simulink model "Mangnorondung"  (R2022b)
settings: Solver=FixedStepAuto  StartTime=0.0  StopTime=150  FixedStep=0.01  RelTol=1e-3
libraries: slpidlib x2
settings Model: Creator=vudin  LastModifiedBy=Acer Nitro
settings SolverCC: ShapePreserveControl=EnableAll  AlgebraicLoopSolver=TrustRegion
settings DataIOCC: ReturnWorkspaceOutputs=off
settings DebuggingCC: UnconnectedInputMsg=warning  UnconnectedOutputMsg=warning  UnconnectedLineMsg=warning  SFMachineParentedDataDiag=warning  ArithmeticOperatorsInVariantConditions=warning
settings ModelReferenceCC: EnableRefExpFcnMdlSchedulingChecks=on
settings SFSimCC: CustomCodeUndefinedFunction=UseInterfaceOnly

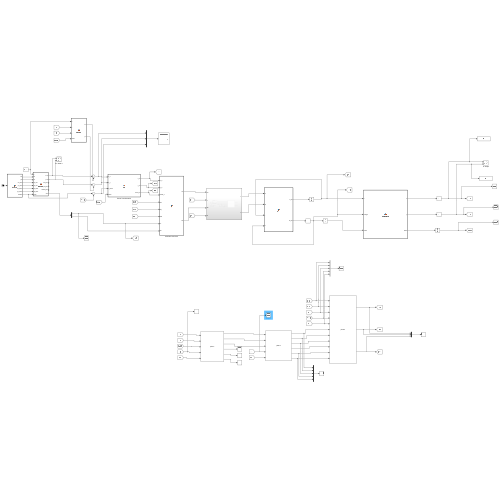
[thumbnail: Simulink's stored preview of the top-level diagram]
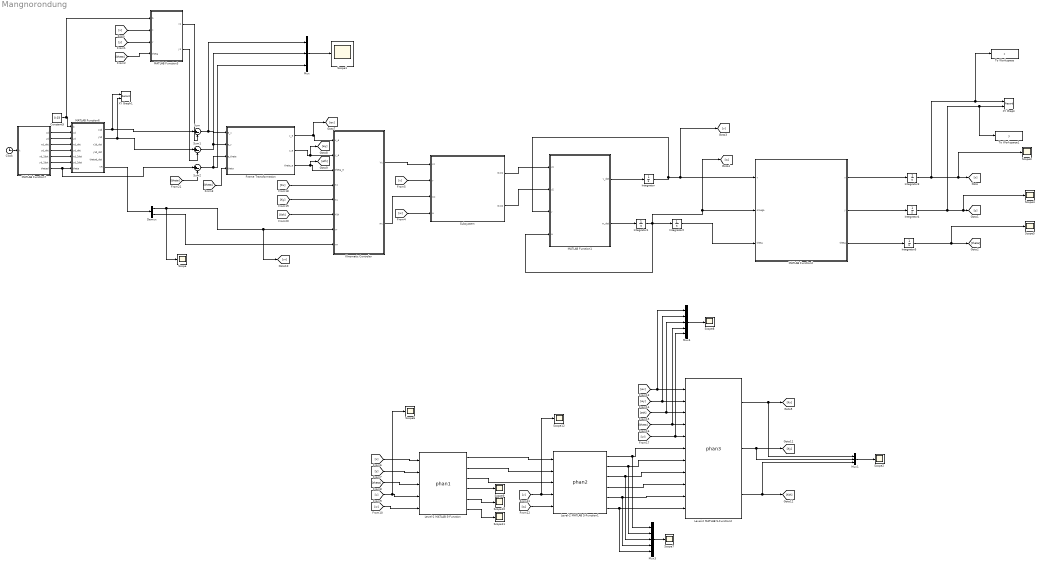
== system Mangnorondung ==
  Clock : Clock
  Constant5 : Constant  Value=0.03
  Demux : Demux  Outputs=2
  Frame Transformation : MATLAB Function  TreatAsAtomicUnit=on
  Integrator{,1..5} (6 alike) : Integrator
  KInematic Controler : MATLAB Function  TreatAsAtomicUnit=on
  Level-2 MATLAB S-Function : M-S-Function  FunctionName=phan1
  Level-2 MATLAB S-Function1 : M-S-Function  FunctionName=phan2
  Level-2 MATLAB S-Function2 : M-S-Function  FunctionName=phan3
  MATLAB Function1 : MATLAB Function  TreatAsAtomicUnit=on
  MATLAB Function2 : MATLAB Function  TreatAsAtomicUnit=on
  MATLAB Function3 : MATLAB Function  TreatAsAtomicUnit=on
  MATLAB Function6 : MATLAB Function  TreatAsAtomicUnit=on
  MATLAB Function7 : MATLAB Function  TreatAsAtomicUnit=on
  Mux : Mux  Inputs=3
  Mux1 : Mux  Inputs=3
  Mux3 : Mux  Inputs=5
  Mux4 : Mux  Inputs=5
  Scope{,1..12} (13 alike) : Scope
  Subsystem : Subsystem
  Sum : Sum  Inputs=|+-
  Sum1 : Sum  Inputs=|+-
  Sum2 : Sum  Inputs=|+-
  To Workspace : ToWorkspace  VariableName=x  SampleTime=-1
  To Workspace1 : ToWorkspace  VariableName=y  SampleTime=-1
  XY Graph : Record  FileSettingsInternal="{\"entries\":[{\"content\":{\"excelSettings\":{\"content\":{},\"type\":\"Streamout.ExcelSettings\"}},\"type\":\"Streamout.FileSettingStorage\",\"uuid\":\"709517b4-b6f2-4336-ad97-cda2d1ea3157\"}],\"packageUris\":[\"http://schema.mathworks.com/mf0/streamout_blocks/R2020a\"],\"version\":\"1.0\"}"  Layout=[1 1]  SignalsInternal="{\"entries\":[{\"content\":{\"signals\":[{\"content\":{\"blockPath\":[\"Mangnorondung/XY Graph\"],\"channel\":[],\"dimensions\":[1],\"domain\":\"Mangnorondung/XY Graph\",\"lineColor\":\"#a2142f\",\"plots\":[1],\"port\":1,\"sid\":[\"\"],\"signalID\":43589,\"signalName\":\"Integrator3\"},\"type\":\"RecordBlkView.Signal\",\"uuid\":\"4f684b5a-924f-486e-9d40-9f936f114ddd\"},{\"content\":{\"blockPath\":[\"Mangnorondung/XY Graph\"],\"channel\":[],\"dimensions\":[1],\"domain\":\"Mangnorondung/XY Graph\",\"lineColor\":\"#139fff\",\"plots\":[1],\"port\":2,\"sid\":[\"\"],\"signalID\":43593,\"signalName\":\"Integrator4\"},\"type\":\"RecordBlkView.Signal\",\"uuid\":\"4d6a86e3-ef4b-4abf-8449-7e6d24bf3609\"}]},\"type\":\"RecordBlkView.InputSignals\",\"uuid\":\"2b587b06-57ab-4d61-b86d-7002576b861b\"}],\"packageUris\":[\"http://schema.mathworks.com/mf0/streamout_blocks/R2020a\"],\"version\":\"1.0\"}"  VisualizationBindings="{\"xyplotplugin\":{\"info\":[{\"series\":[{\"bindingParametersList\":[{\"parameter\":\"X-Axis\",\"signalID\":43589,\"signalName\":\"Integrator3\"},{\"parameter\":\"Y-Axis\",\"signalID\":43593,\"signalName\":\"Integrator4\"}],\"seriesID\":42575}],\"subplotID\":1}]}}"  CompatibilityTag=XY  st=-1
  XY Graph1 : Record  FileSettingsInternal="{\"entries\":[{\"content\":{\"excelSettings\":{\"content\":{},\"type\":\"Streamout.ExcelSettings\"}},\"type\":\"Streamout.FileSettingStorage\",\"uuid\":\"df5eb68b-e3d3-4db8-aae6-13adc78e2c49\"}],\"packageUris\":[\"http://schema.mathworks.com/mf0/streamout_blocks/R2020a\"],\"version\":\"1.0\"}"  Layout=[1 1]  SignalsInternal="{\"entries\":[{\"content\":{\"signals\":[{\"content\":{\"blockPath\":[\"Mangnorondung/XY Graph1\"],\"channel\":[],\"dimensions\":[1],\"domain\":\"Mangnorondung/XY Graph1\",\"lineColor\":\"#a2142f\",\"plots\":[1],\"port\":1,\"sid\":[\"\"],\"signalID\":43597,\"signalName\":\"MATLAB Function6:1\"},\"type\":\"RecordBlkView.Signal\",\"uuid\":\"7454b842-5480-4a32-880b-5852a87a060b\"},{\"content\":{\"blockPath\":[\"Mangnorondung/XY Graph1\"],\"channel\":[],\"dimensions\":[1],\"domain\":\"Mangnorondung/XY Graph1\",\"lineColor\":\"#139fff\",\"plots\":[1],\"port\":2,\"sid\":[\"\"],\"signalID\":43601,\"signalName\":\"MATLAB Function6:2\"},\"type\":\"RecordBlkView.Signal\",\"uuid\":\"a917114d-4933-41c9-b594-8cfc2867815e\"}]},\"type\":\"RecordBlkView.InputSignals\",\"uuid\":\"cfe23017-764e-4c0d-8e92-bd75a684a487\"}],\"packageUris\":[\"http://schema.mathworks.com/mf0/streamout_blocks/R2020a\"],\"version\":\"1.0\"}"  VisualizationBindings="{\"xyplotplugin\":{\"info\":[{\"series\":[{\"bindingParametersList\":[{\"parameter\":\"X-Axis\",\"signalID\":43597,\"signalName\":\"MATLAB Function6:1\"},{\"parameter\":\"Y-Axis\",\"signalID\":43601,\"signalName\":\"MATLAB Function6:2\"}],\"seriesID\":38209}],\"subplotID\":1}]}}"  CompatibilityTag=XY  st=-1
  wires:
  Subsystem/1(Out1) -> MATLAB Function1/1(u1)
  MATLAB Function6/1(x1d) -> XY Graph1/1, Sum/1
  Demux/1 -> Scope/1, [vr], KInematic Controler/7(vr)
  Subsystem/2(Out2) -> MATLAB Function1/2(u2)
  MATLAB Function1/1(v_dot) -> Integrator/1
  MATLAB Function6/6(VR) -> Demux/1
  Mux/1 -> Scope1/1
  MATLAB Function2/3(theta) -> Integrator5/1
  Sum2/1 -> Mux/3, Frame Transformation/3(e_theta)
  Integrator2/1 -> MATLAB Function2/3("theta ")
  MATLAB Function2/1(x) -> Integrator3/1
  Integrator5/1 -> Scope5/1, [theta]
  Integrator1/1 -> [w], MATLAB Function2/2(omega), Integrator2/1, MATLAB Function1/4(w)
  MATLAB Function7/6(yd_2dot) -> MATLAB Function6/7(yd_2dot)
  MATLAB Function7/5(xd_2dot) -> MATLAB Function6/6(xd_2dot)
  Frame Transformation/1(x_e) -> [ex], KInematic Controler/1(x_e)
  [v] -> Subsystem/2(v)
  KInematic Controler/1(Vc) -> Subsystem/1(Vc)
  KInematic Controler/2(wc) -> Subsystem/3(wc)
  MATLAB Function2/2(y) -> Integrator4/1
  Constant5/1 -> MATLAB Function3/1(b), MATLAB Function6/1(b)
  Sum/1 -> Frame Transformation/1(e_x), Mux/1
  MATLAB Function7/1(xd) -> MATLAB Function6/2(xd)
  Demux/2 -> KInematic Controler/8(wr)
  Integrator4/1 -> To Workspace1/1, XY Graph/2, Scope4/1, [y]
  MATLAB Function3/2(y1) -> Sum1/2
  Frame Transformation/2(y_e) -> [ey], KInematic Controler/2(y_e)
  Frame Transformation/3(theta_e) -> [eth], KInematic Controler/3(theta_e)
  [x] -> MATLAB Function3/2(x)
  Integrator3/1 -> To Workspace/1, XY Graph/1, Scope3/1, [x]
  Sum1/1 -> Frame Transformation/2(e_y), Mux/2
  MATLAB Function3/1(x1) -> Sum/2
  Clock/1 -> MATLAB Function7/1(t)
  MATLAB Function7/7(thetad) -> Sum2/1, MATLAB Function6/8(theta)
  [y] -> MATLAB Function3/3(y)
  Integrator/1 -> MATLAB Function1/3(v), [v], MATLAB Function2/1(v)
  MATLAB Function7/4(yd_dot) -> MATLAB Function6/5(yd_dot)
  [theta] -> Frame Transformation/4(theta)
  MATLAB Function7/2(yd) -> MATLAB Function6/3(yd)
  [w] -> Subsystem/4(w)
  MATLAB Function1/2(w_dot) -> Integrator1/1
  MATLAB Function6/2(y1d) -> XY Graph1/2, Sum1/1
  MATLAB Function7/3(xd_dot) -> MATLAB Function6/4(xd_dot)
  Level-2 MATLAB S-Function1/1 -> Mux3/1, Level-2 MATLAB S-Function2/6
  Level-2 MATLAB S-Function1/5 -> Mux3/4, Level-2 MATLAB S-Function2/10
  Level-2 MATLAB S-Function1/3 -> Mux3/3, Level-2 MATLAB S-Function2/8
  Level-2 MATLAB S-Function1/4 -> Level-2 MATLAB S-Function2/9
  Level-2 MATLAB S-Function1/2 -> Mux3/2, Level-2 MATLAB S-Function2/7
  Level-2 MATLAB S-Function/3 -> Level-2 MATLAB S-Function1/3
  Level-2 MATLAB S-Function/2 -> Level-2 MATLAB S-Function1/2
  Level-2 MATLAB S-Function/4 -> Scope9/1
  Level-2 MATLAB S-Function/1 -> Level-2 MATLAB S-Function1/1
  Level-2 MATLAB S-Function1/6 -> Mux3/5, Level-2 MATLAB S-Function2/11
  [theta] -> Level-2 MATLAB S-Function/3
  [y] -> Level-2 MATLAB S-Function/2
  [x] -> Level-2 MATLAB S-Function/1
  [v] -> Scope6/1, Level-2 MATLAB S-Function/4
  [w] -> Level-2 MATLAB S-Function/5
  [v] -> Scope12/1, Level-2 MATLAB S-Function1/4
  [w] -> Level-2 MATLAB S-Function1/5
  [ex] -> Mux4/1, Level-2 MATLAB S-Function2/1
  [ey] -> Mux4/2, Level-2 MATLAB S-Function2/2
  [eth] -> Mux4/3, Level-2 MATLAB S-Function2/3
  [theta] -> Mux4/4, Level-2 MATLAB S-Function2/4
  [vr] -> Level-2 MATLAB S-Function2/5, Mux4/5
  Level-2 MATLAB S-Function2/3 -> Mux1/3, [Kth]
  Level-2 MATLAB S-Function2/2 -> Mux1/2, [Ky]
  Level-2 MATLAB S-Function2/1 -> Mux1/1, [Kx]
  Mux1/1 -> Scope2/1
  Mux3/1 -> Scope7/1
  Mux4/1 -> Scope8/1
  [theta] -> MATLAB Function3/4(theta)
  [theta] -> Sum2/2
  [Kx] -> KInematic Controler/4(Kx)
  [Ky] -> KInematic Controler/5(Ky)
  [Kth] -> KInematic Controler/6(Kth)
  Level-2 MATLAB S-Function/5 -> Scope10/1
  Level-2 MATLAB S-Function/6 -> Scope11/1

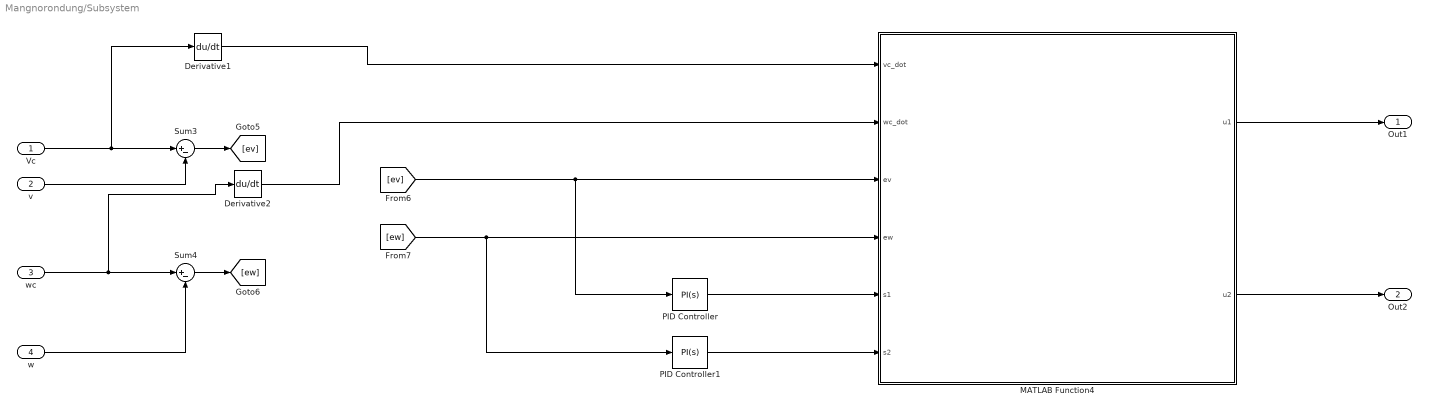
== system Mangnorondung/Subsystem ==
  Vc : Inport
  v : Inport  Port=2
  wc : Inport  Port=3
  w : Inport  Port=4
  Derivative1 : Derivative
  Derivative2 : Derivative
  MATLAB Function4 : MATLAB Function  TreatAsAtomicUnit=on
  PID Controller : slpidlib/PID Controller  Controller=PI  Form=Parallel  TimeDomain=Continuous-time  UseExternalTs=off  SampleTime=-1  IntegratorMethod=Forward Euler  FilterMethod=Forward Euler  ControllerParametersSource=internal  P=1  I=1  UseKiTs=off  D=0  N=100  UseFilter=on  TunerSelectOption=Transfer Function Based (PID Tuner App)  InitialConditionSource=internal  InitialConditionForIntegrator=0  InitialConditionForFilter=0  DifferentiatorICPrevScaledInput=0  ExternalReset=none  TrackingMode=off  Kt=1  LimitOutput=off  SatLimitsSource=internal  UpperSaturationLimit=inf  LowerSaturationLimit=-inf  LinearizeAsGain=on  AntiWindupMode=none  Kb=1  LimitIntegrator=off  UpperIntegratorSaturationLimit=inf  LowerIntegratorSaturationLimit=-inf  POutMin=[]  POutMax=[]  IOutMin=[]  IOutMax=[]  DOutMin=[]  DOutMax=[]  NOutMin=[]  NOutMax=[]  SumOutMin=[]  SumOutMax=[]  SaturationOutMin=[]  SaturationOutMax=[]  PParamMin=[]  PParamMax=[]  IParamMin=[]  IParamMax=[]  DParamMin=[]  DParamMax=[]  NParamMin=[]  NParamMax=[]  KbParamMin=[]  KbParamMax=[]  KtParamMin=[]  KtParamMax=[]  KbOutMin=[]  KbOutMax=[]  KtOutMin=[]  KtOutMax=[]  IntegratorOutMin=[]  IntegratorOutMax=[]  FilterOutMin=[]  FilterOutMax=[]  SumI1OutMin=[]  SumI1OutMax=[]  SumI2OutMin=[]  SumI2OutMax=[]  SumI3OutMin=[]  SumI3OutMax=[]  SumI4OutMin=[]  SumI4OutMax=[]  SumDOutMin=[]  SumDOutMax=[]  DifferentiatorOutMin=[]  DifferentiatorOutMax=[]  FilterDiffOutCoefMin=[]  FilterDiffOutCoefMax=[]  ReciprocalOutMin=[]  ReciprocalOutMax=[]  SumDenOutMin=[]  SumDenOutMax=[]  SumNumOutMin=[]  SumNumOutMax=[]  DivideOutMin=[]  DivideOutMax=[]  UdiffTsProdOutMin=[]  UdiffTsProdOutMax=[]  NTsProdOutMin=[]  NTsProdOutMax=[]  UintegralTsProdOutMin=[]  UintegralTsProdOutMax=[]  UngainTsProdOutMin=[]  UngainTsProdOutMax=[]  ClampingZeroOutDataTypeStr=Inherit: Inherit via back propagation  ClampingZeroOutMin=[]  ClampingZeroOutMax=[]  FilterDenConstantOutDataTypeStr=Inherit: Inherit via back propagation  FilterDenConstantOutMin=[]  FilterDenConstantOutMax=[]  PCopyOutDataTypeStr=Inherit: Inherit via back propagation  PCopyOutMin=[]  PCopyOutMax=[]  NCopyOutDataTypeStr=Inherit: Inherit via back propagation  NCopyOutMin=[]  NCopyOutMax=[]  IntegratorContinuousStateAttributes=''  IntegratorStateMustResolveToSignalObject=off  IntegratorRTWStateStorageClass=Auto  FilterContinuousStateAttributes=''  FilterStateMustResolveToSignalObject=off  FilterRTWStateStorageClass=Auto  ParallelPVariant=InternalParameters  IdealPVariant=Disabled  IVariant=InternalParameters  DVariant=Disabled  IntegratorVariant=Continuous  SatVariant=Disabled  AWVariant=Passthrough  PCopyVariant=Disabled  TRVariant=Disabled  FdbkBlocksVariant=Forward  IdealPFdbkVariant=Disabled  SatFdbkVariant=Disabled  DerivativeFilterVariant=Disabled  NVariant=Disabled  NCopyVariant=Disabled_SignalSpec  FilterICVariant=Disabled  IntegratorICVariant=InternalICs  ExternalResetVariant=Disabled  TRSumVariant=Passthrough  SumFdbkVariant=Disabled  SumVariant=Sum_PI  TsampFilterVariant=InternalTs  TsampNgainVariant=Passthrough  TsampIntegralVariant=Passthrough  ExternalSaturationOutDataTypeStr=Inherit: Same as second input
  PID Controller1 : slpidlib/PID Controller  Controller=PI  Form=Parallel  TimeDomain=Continuous-time  UseExternalTs=off  SampleTime=-1  IntegratorMethod=Forward Euler  FilterMethod=Forward Euler  ControllerParametersSource=internal  P=1  I=1  UseKiTs=off  D=0  N=100  UseFilter=on  TunerSelectOption=Transfer Function Based (PID Tuner App)  InitialConditionSource=internal  InitialConditionForIntegrator=0  InitialConditionForFilter=0  DifferentiatorICPrevScaledInput=0  ExternalReset=none  TrackingMode=off  Kt=1  LimitOutput=off  SatLimitsSource=internal  UpperSaturationLimit=inf  LowerSaturationLimit=-inf  LinearizeAsGain=on  AntiWindupMode=none  Kb=1  LimitIntegrator=off  UpperIntegratorSaturationLimit=inf  LowerIntegratorSaturationLimit=-inf  POutMin=[]  POutMax=[]  IOutMin=[]  IOutMax=[]  DOutMin=[]  DOutMax=[]  NOutMin=[]  NOutMax=[]  SumOutMin=[]  SumOutMax=[]  SaturationOutMin=[]  SaturationOutMax=[]  PParamMin=[]  PParamMax=[]  IParamMin=[]  IParamMax=[]  DParamMin=[]  DParamMax=[]  NParamMin=[]  NParamMax=[]  KbParamMin=[]  KbParamMax=[]  KtParamMin=[]  KtParamMax=[]  KbOutMin=[]  KbOutMax=[]  KtOutMin=[]  KtOutMax=[]  IntegratorOutMin=[]  IntegratorOutMax=[]  FilterOutMin=[]  FilterOutMax=[]  SumI1OutMin=[]  SumI1OutMax=[]  SumI2OutMin=[]  SumI2OutMax=[]  SumI3OutMin=[]  SumI3OutMax=[]  SumI4OutMin=[]  SumI4OutMax=[]  SumDOutMin=[]  SumDOutMax=[]  DifferentiatorOutMin=[]  DifferentiatorOutMax=[]  FilterDiffOutCoefMin=[]  FilterDiffOutCoefMax=[]  ReciprocalOutMin=[]  ReciprocalOutMax=[]  SumDenOutMin=[]  SumDenOutMax=[]  SumNumOutMin=[]  SumNumOutMax=[]  DivideOutMin=[]  DivideOutMax=[]  UdiffTsProdOutMin=[]  UdiffTsProdOutMax=[]  NTsProdOutMin=[]  NTsProdOutMax=[]  UintegralTsProdOutMin=[]  UintegralTsProdOutMax=[]  UngainTsProdOutMin=[]  UngainTsProdOutMax=[]  ClampingZeroOutDataTypeStr=Inherit: Inherit via back propagation  ClampingZeroOutMin=[]  ClampingZeroOutMax=[]  FilterDenConstantOutDataTypeStr=Inherit: Inherit via back propagation  FilterDenConstantOutMin=[]  FilterDenConstantOutMax=[]  PCopyOutDataTypeStr=Inherit: Inherit via back propagation  PCopyOutMin=[]  PCopyOutMax=[]  NCopyOutDataTypeStr=Inherit: Inherit via back propagation  NCopyOutMin=[]  NCopyOutMax=[]  IntegratorContinuousStateAttributes=''  IntegratorStateMustResolveToSignalObject=off  IntegratorRTWStateStorageClass=Auto  FilterContinuousStateAttributes=''  FilterStateMustResolveToSignalObject=off  FilterRTWStateStorageClass=Auto  ParallelPVariant=InternalParameters  IdealPVariant=Disabled  IVariant=InternalParameters  DVariant=Disabled  IntegratorVariant=Continuous  SatVariant=Disabled  AWVariant=Passthrough  PCopyVariant=Disabled  TRVariant=Disabled  FdbkBlocksVariant=Forward  IdealPFdbkVariant=Disabled  SatFdbkVariant=Disabled  DerivativeFilterVariant=Disabled  NVariant=Disabled  NCopyVariant=Disabled_SignalSpec  FilterICVariant=Disabled  IntegratorICVariant=InternalICs  ExternalResetVariant=Disabled  TRSumVariant=Passthrough  SumFdbkVariant=Disabled  SumVariant=Sum_PI  TsampFilterVariant=InternalTs  TsampNgainVariant=Passthrough  TsampIntegralVariant=Passthrough  ExternalSaturationOutDataTypeStr=Inherit: Same as second input
  Sum3 : Sum  Inputs=|+-
  Sum4 : Sum  Inputs=|+-
  Out1 : Outport  VectorParamsAs1DForOutWhenUnconnected=off
  Out2 : Outport  Port=2  VectorParamsAs1DForOutWhenUnconnected=off
  wires:
  Derivative2/1 -> MATLAB Function4/2(wc_dot)
  MATLAB Function4/2(u2) -> Out2/1
  PID Controller1/1 -> MATLAB Function4/6(s2)
  wc/1 -> Derivative2/1, Sum4/1
  PID Controller/1 -> MATLAB Function4/5(s1)
  [ev] -> PID Controller/1, MATLAB Function4/3(ev)
  Sum4/1 -> [ew]
  [ew] -> PID Controller1/1, MATLAB Function4/4(ew)
  w/1 -> Sum4/2
  v/1 -> Sum3/2
  Vc/1 -> Derivative1/1, Sum3/1
  Sum3/1 -> [ev]
  MATLAB Function4/1(u1) -> Out1/1
  Derivative1/1 -> MATLAB Function4/1(vc_dot)

== matlab function Mangnorondung/Subsystem/MATLAB Function4 ==
  data: vc_dot input; u1 output; wc_dot input; ev input; ew input; u2 output; s1 input; s2 input
function [u1,u2] = fcn(vc_dot,wc_dot,ev,ew,s1,s2)
R=0.095;%bánh kính bánh xe
L=0.24; %khoảng cách từ tâm bánh đến tâm DDMR
Iw=0.0023; %momen quán tính của bánh xe dẫn động với bộ truyền động quanh trục bánh xe
mc=17; %khối lượng khi không có bánh và bộ truyền động
mw=0.5; %khối lượng mỗi bánh bao gồm cả hệ truyền động
d=0.05; %khoảng cách giữa điểm gốc và khối tâm
Ic=0.537; %mn quomeán tính của robot với trục xr đi qua tâm
Im=0.0011; %momen quán tính mỗi bánh dẫn động 

m=mc + 2*mw;
I= Ic+ mc*d^2 +2*mw*L^2 +2*Im;
m0= m + (2*Iw)/R^2;
i0= I + (2*L^2*Iw)/R^2;


u1=(vc_dot + 50*ev)*m0*R+0.171*sign(s1);
u2=(wc_dot + 50*ew)*i0*R/L+0.171*sign(s2);

== matlab function Mangnorondung/MATLAB Function7 ==
  data: t input; xd output; yd output; xd_dot output; yd_dot output; xd_2dot output; yd_2dot output; thetad output
function [xd,yd,xd_dot,yd_dot,xd_2dot,yd_2dot,thetad] = quydao(t)
%% Khoi tao quy dao chuyen dong
R=3; %ban kinh quy dao
w=0.1; %rad/s =2*pi*f f=w/2/pi -> T=1/f
xd=R*cos(w*t);
yd=R*sin(w*t);
xd_dot=-R*w*sin(w*t);
yd_dot=R*w*cos(w*t);
x0d_dot=-R*w*sin(w);
y0d_dot=R*w*cos(w);
xd_2dot=-R*w^2*cos(w*t);
yd_2dot=-R*w^2*sin(w*t);
theta0=atan2(y0d_dot,x0d_dot)-w;
thetad=w*t + theta0;

== matlab function Mangnorondung/Frame Transformation ==
  data: e_x input; x_e output; e_y input; e_theta input; y_e output; theta_e output; theta input
function [x_e,y_e,theta_e] = fcn(e_x,e_y,e_theta,theta)
A=[cos(theta) sin(theta) 0;-sin(theta) cos(theta) 0;0 0 1];
B=[e_x;e_y;e_theta];
C=A*B;
x_e=C(1);
y_e=C(2);
theta_e=C(3);
% công thức 45

== matlab function Mangnorondung/KInematic Controler ==
  data: x_e input; Vc output; y_e input; theta_e input; Kx input; Ky input; Kth input; wc output; vr input; wr input
function [Vc,wc] = fcn(x_e,y_e,theta_e,Kx,Ky,Kth,vr,wr)
Vc=vr*cos(theta_e)+ Kx*x_e;
wc=wr+vr*(Ky*y_e + Kth*sin(theta_e));

%công thức 46

== matlab function Mangnorondung/MATLAB Function3 ==
  data: b input; x1 output; y1 output; x input; y input; theta input
function [x1,y1] = quydao(b,x,y,theta)
%% Thiet lap quy dao chuyen dong cho robot
%theta=atan2(yd_dot,xd_dot);
x1=x+b*cos(theta);
y1=y+b*sin(theta);

== matlab function Mangnorondung/MATLAB Function1 ==
  data: u1 input; v_dot output; u2 input; v input; w input; w_dot output
function [v_dot,w_dot]=fcn(u1,u2,v,w)
R=0.095;%bánh kính bánh xe
L=0.24; %khoảng cách từ tâm bánh đến tâm DDMR
Iw=0.0023; %momen quán tính của bánh xe dẫn động với bộ truyền động quanh trục bánh xe
mc=17; %khối lượng khi không có bánh và bộ truyền động
mw=0.5; %khối lượng mỗi bánh bao gồm cả hệ truyền động
d=0.05; %khoảng cách giữa điểm gốc và khối tâm
Ic=0.537; %momen quán tính của robot với trục xr đi qua tâm
Im=0.0011; %momen quán tính mỗi bánh dẫn động 

m=mc + 2*mw;
I= Ic+ mc*d^2 +2*mw*L^2 +2*Im;
m0= m + (2*Iw)/R^2;
i0= I + (2*L^2*Iw)/R^2;

M=[m0 0;0 i0];
V=[0 -mc*d*w;mc*d*w 0];
T=[1/R 0;0 L/R];
u=[u1;u2];
k=[v;w];

N=T*u-V*k;
Z=inv(M)*N;
v_dot=Z(1);
w_dot=Z(2);

== matlab function Mangnorondung/MATLAB Function2 ==
  data: v input; x output; omega input; theta input; y output; theta output
function [x,y,theta]=Kinematics(v,omega,theta)

S=[cos(theta) 0;
 sin(theta) 0;
 0 1];
ve=[v;omega];
qdot=S*ve;
x=qdot(1);

y=qdot(2);
theta=qdot(3);

== matlab function Mangnorondung/MATLAB Function6 ==
  data: b input; x1d output; y1d output; x1d_dot output; y1d_dot output; thetad_dot output; xd input; yd input; xd_dot input; yd_dot input; xd_2dot input; yd_2dot input; theta input; VR output
function [x1d,y1d,x1d_dot,y1d_dot,thetad_dot,VR] = quydao(b,xd,yd,xd_dot,yd_dot,xd_2dot,yd_2dot,theta)
%% Thiet lap quy dao chuyen dong cho robot
%theta=atan2(yd_dot,xd_dot);
x1d=xd+b*cos(theta);
y1d=yd+b*sin(theta);
wd=(yd_2dot*xd_dot - xd_2dot*yd_dot)/(xd_dot^2+yd_dot^2);
x1d_dot=xd_dot-b*wd*sin(theta);
y1d_dot=yd_dot+b*wd*cos(theta);
thetad_dot=wd;
rot=[cos(theta) 0; sin(theta) 0; 0 1];
p_dot=[xd_dot; yd_dot; wd];
VR=rot\p_dot;
